simulink model "ABS"  (R2025a)
settings: Solver=ode3  StartTime=0.0  StopTime=8.0  FixedStep=0.001  RelTol=1e-3
model workspace (MAT data in the model file):
  ABS_mode = 1
  ABS_off = 0
  ABS_on = 1
  C = 0.55
  I = 5
  PBmax = 15
  Re = 0.01
  Rw = 0.33415
  force_scaling = 2000
  g = 9.81
  m = 1100
  mu = [0 0.0789791761613 0.156696659243 0.231962689784 0.303722938599 0.371106774378 0.433456326688 0.490335596383 0.541521733827 0.586982573793 0.626845384878 0.661361672136 0.690872066436 0.715774196452 0.736495269686 0.753470085089 0.767124453289 0.777863521405 0.786064249582 0.792071207239 0.796194889632 0.798711850307 0.799866066279 0.799871076669 0.798912548688 0.797151020886 0.794724651039 0.791751855829 0.788333774034 0.784556516974 0.780493192225 0.776205701359 0.77174632185 0.767159088641 0.762480993606 0.757743021983 0.752971044565 0.748186583428 0.743407467535 0.73864839302 0.733921401283 0.729236286485 0.724600942561 0.720021658523 0.715503369616 0.711049870856 0.706663998509 0.702347784291 0.698102586355 0.693929200534 0.689827954784 0.685798789352 0.681841324785 0.677954919605 0.674138719194 0.670391697183 0.666712690484 0.663100428882 0.659553560022 0.656070670452 0.652650303317 0.649290973205 0.645991178554 0.642749411996 0.639564168931 0.636433954611 0.633357289934 0.630332716168 0.627358798746 0.624434130277 0.621557332899 0.618727060072 0.615941997892 0.613200866015 0.610502418237 0.6078454428 0.605228762461 0.602651234366 0.600111749767 0.597609233609 0.595142644 0.592710971612 0.590313238998 0.587948499872 0.585615838334 0.583314368082 0.581043231591 0.578801599291 0.576588668734 0.57440366376 0.572245833677 0.570114452435 0.568008817826 0.565928250691 0.563872094137 0.561839712788 0.559830492034 0.557843837318 0.555879173433 0.553935943838]
  slip = [0 0.010101010101 0.020202020202 0.030303030303 0.040404040404 0.0505050505051 0.0606060606061 0.0707070707071 0.0808080808081 0.0909090909091 0.10101010101 0.111111111111 0.121212121212 0.131313131313 0.141414141414 0.151515151515 0.161616161616 0.171717171717 0.181818181818 0.191919191919 0.20202020202 0.212121212121 0.222222222222 0.232323232323 0.242424242424 0.252525252525 0.262626262626 0.272727272727 0.282828282828 0.292929292929 0.30303030303 0.313131313131 0.323232323232 0.333333333333 0.343434343434 0.353535353535 0.363636363636 0.373737373737 0.383838383838 0.393939393939 0.40404040404 0.414141414141 0.424242424242 0.434343434343 0.444444444444 0.454545454545 0.464646464646 0.474747474747 0.484848484848 0.494949494949 0.505050505051 0.515151515152 0.525252525253 0.535353535354 0.545454545455 0.555555555556 0.565656565657 0.575757575758 0.585858585859 0.59595959596 0.606060606061 0.616161616162 0.626262626263 0.636363636364 0.646464646465 0.656565656566 0.666666666667 0.676767676768 0.686868686869 0.69696969697 0.707070707071 0.717171717172 0.727272727273 0.737373737374 0.747474747475 0.757575757576 0.767676767677 0.777777777778 0.787878787879 0.79797979798 0.808080808081 0.818181818182 0.828282828283 0.838383838384 0.848484848485 0.858585858586 0.868686868687 0.878787878788 0.888888888889 0.89898989899 0.909090909091 0.919191919192 0.929292929293 0.939393939394 0.949494949495 0.959595959596 0.969696969697 0.979797979798 0.989898989899 1]
  torque_scaling = 2000
  v0 = 32
libraries: simulink x1
settings Model: Creator=howardchueh  LastModifiedBy=howardchueh

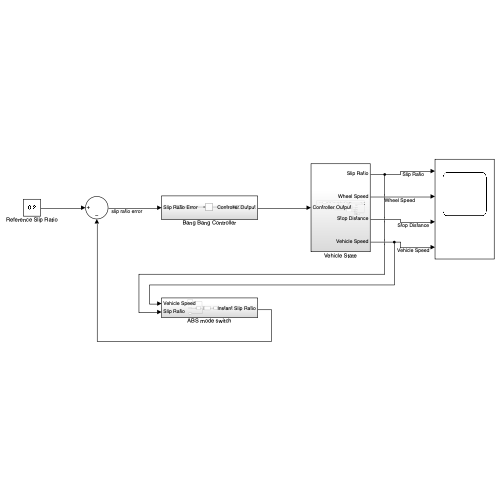
[thumbnail: Simulink's stored preview of the top-level diagram]
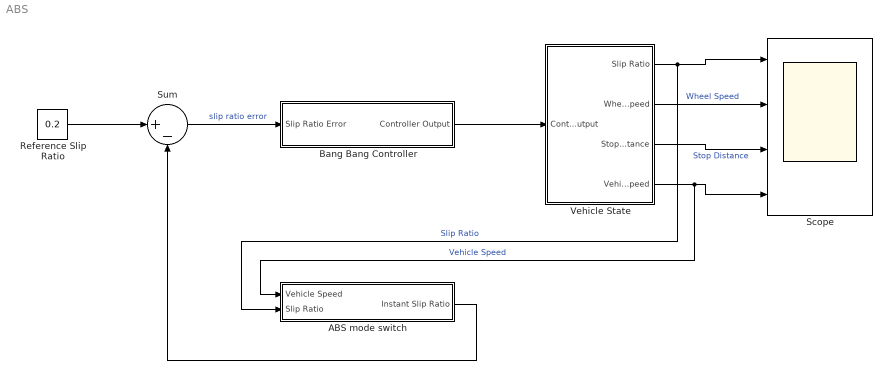
== system ABS ==
  ABS mode switch : Subsystem
  Bang Bang Controller : Subsystem
  Reference Slip Ratio : Constant  Value=0.2
  Scope : Scope  NumInputPorts=4
      settings: ActiveDisplayYMinimum=-1.5591608374452872  ActiveDisplayYMaximum=1.2843512041605873
  Sum : Sum  Inputs=|+-
  Vehicle State : Subsystem
  wires:
  Reference Slip Ratio/1 -> Sum/1
  Sum/1 -> Bang Bang Controller/1(Slip Ratio Error)  "slip ratio error"
  ABS mode switch/1(Instant Slip Ratio) -> Sum/2
  Bang Bang Controller/1(Controller Output) -> Vehicle State/1(Controller Output)
  Vehicle State/1(Slip Ratio) -> Scope/1, ABS mode switch/2(Slip Ratio)  "Slip Ratio"
  Vehicle State/2(Wheel Speed) -> Scope/2  "Wheel Speed"
  Vehicle State/3(Stop Distance) -> Scope/3  "Stop Distance"
  Vehicle State/4(Vehicle Speed) -> Scope/4, ABS mode switch/1(Vehicle Speed)  "Vehicle Speed"

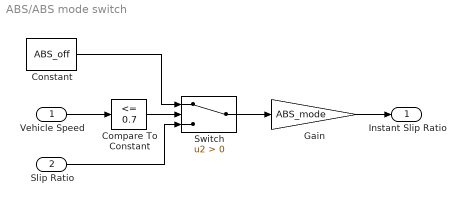
== system ABS/ABS mode switch ==
  Vehicle Speed : Inport
  Slip Ratio : Inport  Port=2
  Compare To Constant : simulink/Logic and Bit Operations/Compare To Constant  relop=<=  const=0.7  OutDataTypeStr=boolean
  Constant : Constant  Value=ABS_off
  Gain : Gain  Gain=ABS_mode
  Switch : Switch  Criteria=u2 > Threshold  SaturateOnIntegerOverflow=off  InputSameDT=off
  Instant Slip Ratio : Outport
  wires:
  Vehicle Speed/1 -> Compare To Constant/1
  Gain/1 -> Instant Slip Ratio/1
  Compare To Constant/1 -> Switch/2
  Constant/1 -> Switch/1
  Slip Ratio/1 -> Switch/3
  Switch/1 -> Gain/1

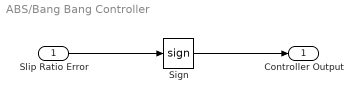
== system ABS/Bang Bang Controller ==
  Slip Ratio Error : Inport
  Sign : Signum
  Controller Output : Outport
  wires:
  Slip Ratio Error/1 -> Sign/1
  Sign/1 -> Controller Output/1

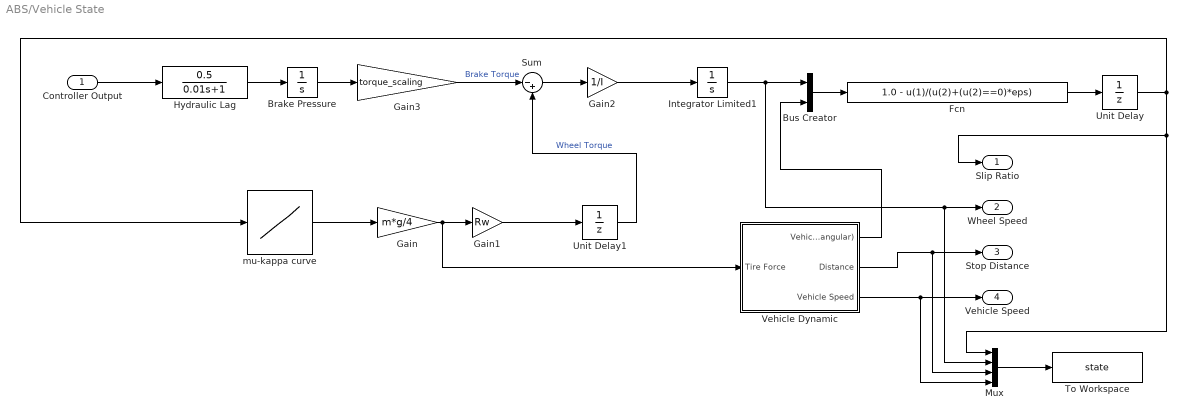
== system ABS/Vehicle State ==
  Controller Output : Inport
  Brake Pressure : Integrator  LimitOutput=on  UpperSaturationLimit=PBmax  LowerSaturationLimit=0
  Bus Creator : BusCreator  Inputs=2
  Fcn : Fcn  Expr=1.0 - u(1)/(u(2)+(u(2)==0)*eps)
  Gain : Gain  Gain=m*g/4
  Gain1 : Gain  Gain=Rw
  Gain2 : Gain  Gain=1/I
  Gain3 : Gain  Gain=torque_scaling
  Hydraulic Lag : TransferFcn  Numerator=[0.5]  Denominator=[0.01 1]
  Integrator Limited1 : Integrator  InitialCondition=v0/Rw  LimitOutput=on  UpperSaturationLimit=100  LowerSaturationLimit=0
  Mux : Mux
  Sum : Sum  Inputs=|-+
  To Workspace : ToWorkspace  VariableName=state  SaveFormat=Timeseries  SampleTime=-1
  Unit Delay : UnitDelay  SampleTime=-1  HasFrameUpgradeWarning=on
  Unit Delay1 : UnitDelay  SampleTime=-1  HasFrameUpgradeWarning=on
  Vehicle Dynamic : Subsystem
  mu-kappa curve : Lookup_n-D  NumberOfTableDimensions=1  BreakpointsForDimension1=slip  Table=mu  InternalRulePriority=Speed  RndMeth=Simplest
  Slip Ratio : Outport
  Wheel Speed : Outport  Port=2
  Stop Distance : Outport  Port=3
  Vehicle Speed : Outport  Port=4
  wires:
  Vehicle Dynamic/3(Vehicle Speed) -> Vehicle Speed/1, Mux/4
  Vehicle Dynamic/2(Distance) -> Stop Distance/1, Mux/3
  Mux/1 -> To Workspace/1
  Gain3/1 -> Sum/1  "Brake Torque"
  Unit Delay1/1 -> Sum/2  "Wheel Torque"
  Sum/1 -> Gain2/1
  Gain2/1 -> Integrator Limited1/1
  Integrator Limited1/1 -> Wheel Speed/1, Mux/2, Bus Creator/1
  Vehicle Dynamic/1(Vehicle Speed (angular)) -> Bus Creator/2
  Bus Creator/1 -> Fcn/1
  Fcn/1 -> Unit Delay/1
  mu-kappa curve/1 -> Gain/1
  Gain/1 -> Vehicle Dynamic/1(Tire Force), Gain1/1
  Gain1/1 -> Unit Delay1/1
  Unit Delay/1 -> Slip Ratio/1, Mux/1, mu-kappa curve/1
  Controller Output/1 -> Hydraulic Lag/1
  Hydraulic Lag/1 -> Brake Pressure/1
  Brake Pressure/1 -> Gain3/1

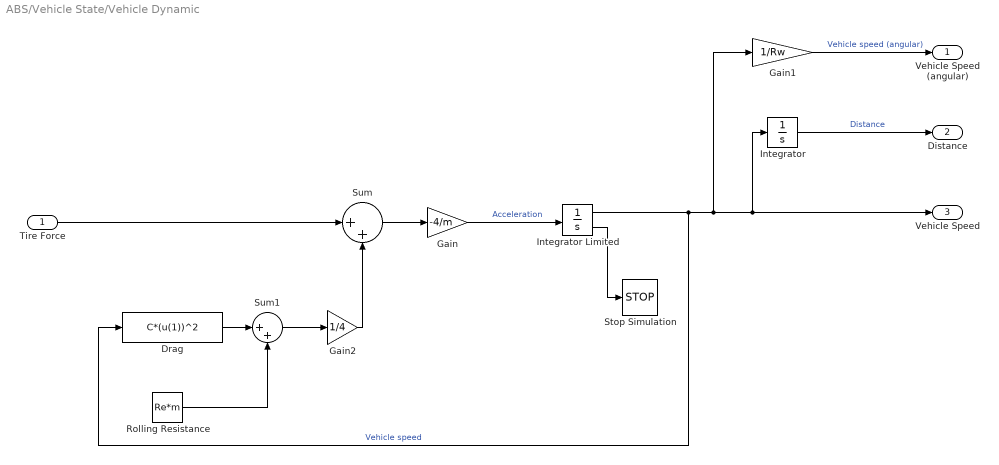
== system ABS/Vehicle State/Vehicle Dynamic ==
  Tire Force : Inport
  Drag : Fcn  Expr=C*(u(1))^2
  Gain : Gain  Gain=-4/m
  Gain1 : Gain  Gain=1/Rw
  Gain2 : Gain  Gain=1/4
  Integrator : Integrator
  Integrator Limited : Integrator  InitialCondition=v0  LimitOutput=on  UpperSaturationLimit=100  LowerSaturationLimit=0  ShowSaturationPort=on
  Rolling Resistance : Constant  Value=Re*m
  Stop Simulation : Stop
  Sum : Sum  Inputs=|++
  Sum1 : Sum  Inputs=|++
  Vehicle Speed (angular) : Outport
  Distance : Outport  Port=2
  Vehicle Speed : Outport  Port=3
  wires:
  Sum1/1 -> Gain2/1
  Rolling Resistance/1 -> Sum1/2
  Integrator Limited/1 -> Drag/1, Gain1/1, Vehicle Speed/1, Integrator/1  "Vehicle speed"
  Gain1/1 -> Vehicle Speed (angular)/1  "Vehicle speed (angular)"
  Drag/1 -> Sum1/1
  Gain2/1 -> Sum/2
  Gain/1 -> Integrator Limited/1  "Acceleration"
  Sum/1 -> Gain/1
  Integrator Limited/2 -> Stop Simulation/1
  Integrator/1 -> Distance/1  "Distance"
  Tire Force/1 -> Sum/1
